simulink model "F_8e"  (R2017a)
settings: Solver=VariableStepAuto  StartTime=0.0  StopTime=50  RelTol=1e-3
undefined symbols (not defined in the file or in its folder): F_animation
libraries: simulink x3
settings Model: Creator=Mat Haskell  LastModifiedBy=Mat Haskell

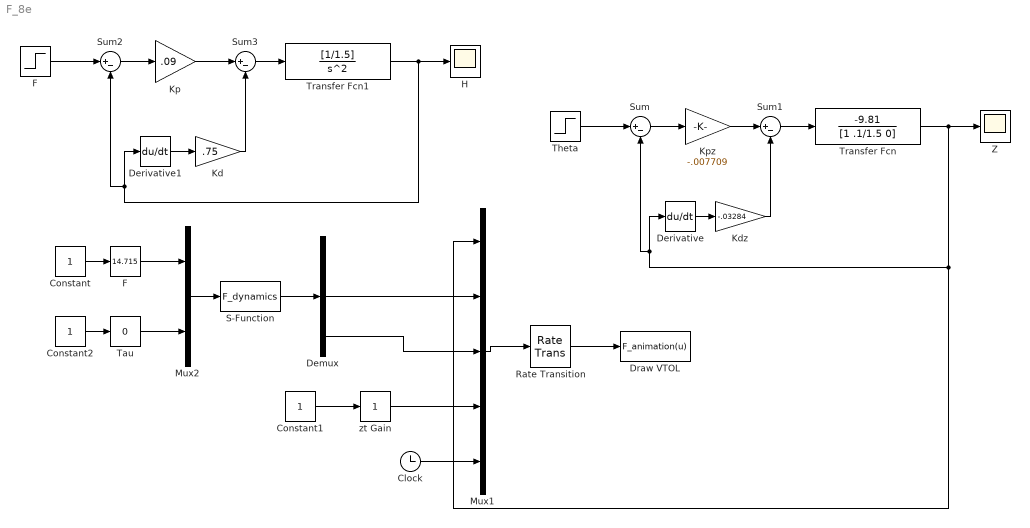
== system F_8e ==
  Clock : Clock
  Constant : Constant
  Constant1 : Constant
  Constant2 : Constant
  Demux : Demux  Outputs=3
  Derivative : Derivative
  Derivative1 : Derivative
  Draw VTOL : MATLABFcn  InitFcn=|  MATLABFcn=F_animation(u)  OutputDimensions=0
      | clear;clc
      | F_param
  F : simulink/Math Operations/Slider Gain  gain=14.715  low=0  high=20
  "F " : Step  SampleTime=0
  "H " : Scope
  "Kd " : Gain  Gain=.75
  "Kdz " : Gain  Gain=-.03284
  Kp : Gain  Gain=.09
  Kpz : Gain  Gain=-.007709
  Mux1 : Mux  Inputs=5
  Mux2 : Mux  Inputs=2
  Rate Transition : RateTransition  OutPortSampleTime=P.t_plot
  S-Function : S-Function  FunctionName=F_dynamics  Parameters=P  SFunctionDeploymentMode=off  EnableBusSupport=off
  Sum{,1..3} (4 alike) : Sum  Inputs=|+-
  Tau : simulink/Math Operations/Slider Gain  gain=0  low=-2  high=2
  "Theta " : Step  SampleTime=0
  Transfer Fcn : TransferFcn  Numerator=[-9.81]  Denominator=[1 .1/1.5 0]
  Transfer Fcn1 : TransferFcn  Numerator=[1/1.5]  Denominator=[1 0 0]
  "Z " : Scope
  zt Gain : simulink/Math Operations/Slider Gain  gain=1  low=0  high=5
  wires:
  "Kdz "/1 -> Sum1/2
  Derivative/1 -> "Kdz "/1
  Sum1/1 -> Transfer Fcn/1
  Sum/1 -> Kpz/1
  Kpz/1 -> Sum1/1
  "Theta "/1 -> Sum/1
  Transfer Fcn/1 -> Mux1/1, Sum/2, Derivative/1, "Z "/1
  F/1 -> Mux2/1
  Constant1/1 -> zt Gain/1
  Mux2/1 -> S-Function/1
  Mux1/1 -> Rate Transition/1
  Constant2/1 -> Tau/1
  Tau/1 -> Mux2/2
  Constant/1 -> F/1
  S-Function/1 -> Demux/1
  Rate Transition/1 -> Draw VTOL/1
  Sum3/1 -> Transfer Fcn1/1
  "Kd "/1 -> Sum3/2
  Kp/1 -> Sum3/1
  Clock/1 -> Mux1/5
  Transfer Fcn1/1 -> Sum2/2, Derivative1/1, "H "/1
  Sum2/1 -> Kp/1
  "F "/1 -> Sum2/1
  zt Gain/1 -> Mux1/4
  Derivative1/1 -> "Kd "/1
  Demux/3 -> Mux1/3
  Demux/2 -> Mux1/2
